simulink model "sliding_control"  (R2013a)
settings: Solver=ode5  StartTime=0.0  StopTime=10.0  FixedStep=0.01  RelTol=1e-3
values from neighbouring files (symbols this model uses):
  epsilon = 0.1    [Hanoi_GUI.m]
  G_T = G'    [Hanoi_GUI.m]
  K = [Kp Kd]    [Hanoi_GUI.m]
  P = lyap(F,eye(4))    [Hanoi_GUI.m]    (also in Lyapunov_P.m)
  U = 0    [Hanoi_GUI.m]
undefined symbols (not defined in the file or in its folder): directhanoi, feedback_lin, hanoidynamics, hanoitraj, inversehanoi
settings Model: Creator=dmar  LastModifiedBy=spaudel

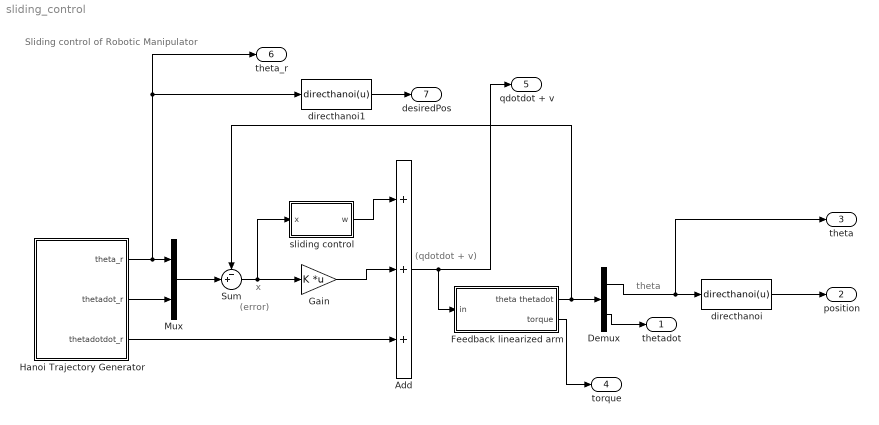
== system sliding_control ==
  note: (error)
  note: (qdotdot + v)
  note: Sliding control of Robotic Manipulator
  note: x
  note: theta
  Add : Sum  Inputs=+++
  Demux : Demux  Outputs=2
  Feedback linearized arm : Subsystem
  Gain : Gain  Gain=K  Multiplication=Matrix(K*u)
  Hanoi Trajectory Generator : Subsystem
  Mux : Mux  Inputs=2
  Sum : Sum  Inputs=-+|
  directhanoi : MATLABFcn  MATLABFcn=directhanoi(u)
  directhanoi1 : MATLABFcn  MATLABFcn=directhanoi(u)
  sliding control : Subsystem
  thetadot : Outport
  position : Outport  Port=2
  theta : Outport  Port=3
  torque : Outport  Port=4
  qdotdot + v : Outport  Port=5
  theta_r : Outport  Port=6
  desiredPos : Outport  Port=7
  wires:
  Hanoi Trajectory Generator/2(thetadot_r) -> Mux/2
  Hanoi Trajectory Generator/1(theta_r) -> directhanoi1/1, theta_r/1, Mux/1
  Sum/1 -> sliding control/1(x), Gain/1
  Feedback linearized arm/1(theta thetadot) -> Demux/1, Sum/1
  Demux/2 -> thetadot/1
  Demux/1 -> theta/1, directhanoi/1
  directhanoi/1 -> position/1
  Feedback linearized arm/2(torque) -> torque/1
  sliding control/1(w) -> Add/1
  Gain/1 -> Add/2
  Hanoi Trajectory Generator/3(thetadotdot_r) -> Add/3
  Add/1 -> qdotdot + v/1, Feedback linearized arm/1(in)
  Mux/1 -> Sum/2
  directhanoi1/1 -> desiredPos/1

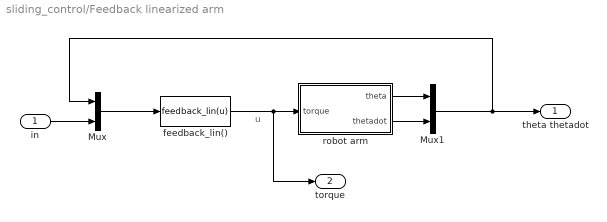
== system sliding_control/Feedback linearized arm ==
  note: u
  in : Inport
  Mux : Mux  Inputs=2
  Mux1 : Mux  Inputs=2
  feedback_lin() : MATLABFcn  MATLABFcn=feedback_lin(u)
  robot arm : Subsystem
  theta thetadot : Outport
  torque : Outport  Port=2
  wires:
  in/1 -> Mux/2
  Mux/1 -> feedback_lin()/1
  feedback_lin()/1 -> torque/1, robot arm/1(torque)
  robot arm/1(theta) -> Mux1/1
  robot arm/2(thetadot) -> Mux1/2
  Mux1/1 -> Mux/1, theta thetadot/1

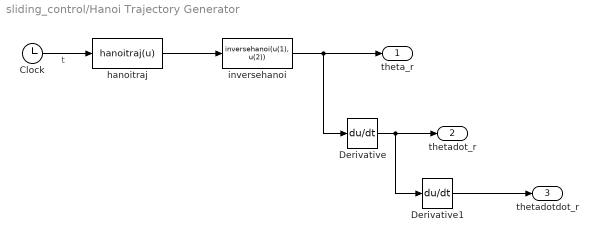
== system sliding_control/Hanoi Trajectory Generator ==
  note: t
  Clock : Clock
  Derivative : Derivative
  Derivative1 : Derivative
  hanoitraj : MATLABFcn  MATLABFcn=hanoitraj(u)
  inversehanoi : MATLABFcn  MATLABFcn=inversehanoi(u(1), u(2))
  theta_r : Outport
  thetadot_r : Outport  Port=2
  thetadotdot_r : Outport  Port=3
  wires:
  hanoitraj/1 -> inversehanoi/1
  Derivative/1 -> thetadot_r/1, Derivative1/1
  inversehanoi/1 -> theta_r/1, Derivative/1
  Clock/1 -> hanoitraj/1
  Derivative1/1 -> thetadotdot_r/1

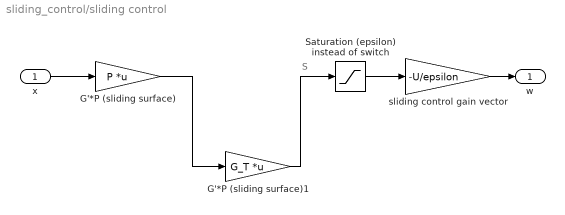
== system sliding_control/sliding control ==
  note: S
  x : Inport
  G'*P (sliding surface) : Gain  Gain=P  Multiplication=Matrix(K*u)
  G'*P (sliding surface)1 : Gain  Gain=G_T  Multiplication=Matrix(K*u)
  Saturation (epsilon) instead of switch : Saturate  UpperLimit=epsilon  LowerLimit=-epsilon
  sliding control gain vector : Gain  Gain=-U/epsilon
  w : Outport
  wires:
  x/1 -> G'*P (sliding surface)/1
  Saturation (epsilon) instead of switch/1 -> sliding control gain vector/1
  sliding control gain vector/1 -> w/1
  G'*P (sliding surface)/1 -> G'*P (sliding surface)1/1
  G'*P (sliding surface)1/1 -> Saturation (epsilon) instead of switch/1

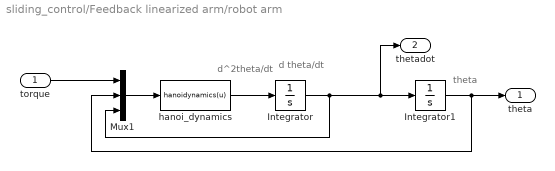
== system sliding_control/Feedback linearized arm/robot arm ==
  note: d^2theta/dt
  note: d theta/dt
  note: theta
  torque : Inport
  Integrator : Integrator  InitialCondition=[0;0]
  Integrator1 : Integrator  InitialCondition=[pi/2;-pi/2]
  Mux1 : Mux  Inputs=3
  hanoi_dynamics : MATLABFcn  MATLABFcn=hanoidynamics(u)
  theta : Outport
  thetadot : Outport  Port=2
  wires:
  hanoi_dynamics/1 -> Integrator/1
  Integrator/1 -> Mux1/3, thetadot/1, Integrator1/1
  Integrator1/1 -> theta/1, Mux1/2
  Mux1/1 -> hanoi_dynamics/1
  torque/1 -> Mux1/1
